simulink model "filter_t1"  (R2017a)
settings: Solver=VariableStepAuto  StartTime=0.0  StopTime=19  RelTol=1e-3
settings Model: Creator=Chaohua Zhao  LastModifiedBy=Chaohua Zhao

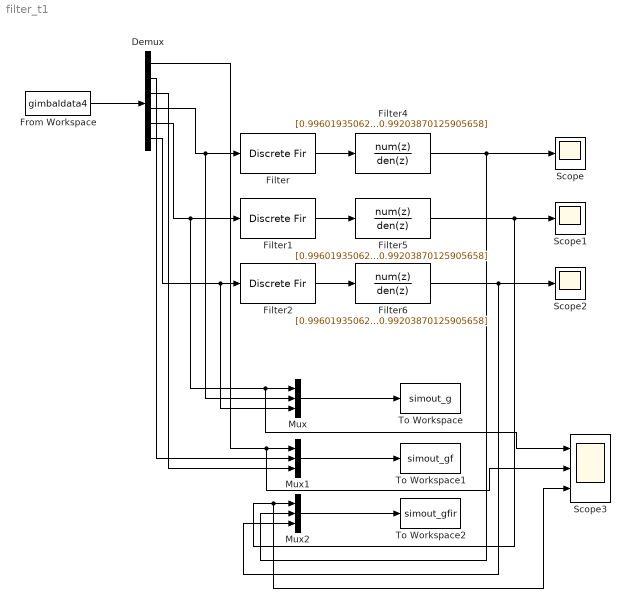
== system filter_t1 ==
  Demux : Demux  Outputs=6
  Filter : DiscreteFir  Tag=BlockMethodSubSystem  Coefficients=[6.3171406458817249e-18 0.038757485800321609 0.085067928451757008 0.12917070559097471 0.16083305039150533 0.17234165953088285 0.16083305039150533 0.12917070559097471 0.085067928451757008 0.038757485800321609 6.3171406458817249e-18]  InputProcessing=Columns as channels (frame based)
  Filter1 : DiscreteFir  Tag=BlockMethodSubSystem  Coefficients=[6.3171406458817249e-18 0.038757485800321609 0.085067928451757008 0.12917070559097471 0.16083305039150533 0.17234165953088285 0.16083305039150533 0.12917070559097471 0.085067928451757008 0.038757485800321609 6.3171406458817249e-18]  InputProcessing=Columns as channels (frame based)
  Filter2 : DiscreteFir  Tag=BlockMethodSubSystem  Coefficients=[6.3171406458817249e-18 0.038757485800321609 0.085067928451757008 0.12917070559097471 0.16083305039150533 0.17234165953088285 0.16083305039150533 0.12917070559097471 0.085067928451757008 0.038757485800321609 6.3171406458817249e-18]  InputProcessing=Columns as channels (frame based)
  Filter4 : DiscreteFilter  Tag=BlockMethodSubSystem  Numerator=[0.99601935062952829 -1.8886556848759783 0.99601935062952829]  Denominator=[1 -1.8886556848759783 0.99203870125905658]  InputProcessing=Columns as channels (frame based)  a0EqualsOne=on
  Filter5 : DiscreteFilter  Tag=BlockMethodSubSystem  Numerator=[0.99601935062952829 -1.8886556848759783 0.99601935062952829]  Denominator=[1 -1.8886556848759783 0.99203870125905658]  InputProcessing=Columns as channels (frame based)  a0EqualsOne=on
  Filter6 : DiscreteFilter  Tag=BlockMethodSubSystem  Numerator=[0.99601935062952829 -1.8886556848759783 0.99601935062952829]  Denominator=[1 -1.8886556848759783 0.99203870125905658]  InputProcessing=Columns as channels (frame based)  a0EqualsOne=on
  From Workspace : FromWorkspace  VariableName=gimbaldata4  SampleTime=0.001  OutputAfterFinalValue=Setting to zero
  Mux : Mux  Inputs=3
  Mux1 : Mux  Inputs=3
  Mux2 : Mux  Inputs=3
  Scope : Scope
  Scope1 : Scope
  Scope2 : Scope
  Scope3 : Scope  NumInputPorts=3
  To Workspace : ToWorkspace  VariableName=simout_g  SampleTime=-1
  To Workspace1 : ToWorkspace  VariableName=simout_gf  SampleTime=-1
  To Workspace2 : ToWorkspace  VariableName=simout_gfir  SampleTime=-1
  wires:
  From Workspace/1 -> Demux/1
  Demux/4 -> Mux/2, Filter/1
  Demux/5 -> Scope3/1, Mux/1, Filter1/1
  Demux/6 -> Mux/3, Filter2/1
  Filter/1 -> Filter4/1
  Filter1/1 -> Filter5/1
  Filter2/1 -> Filter6/1
  Mux/1 -> To Workspace/1
  Demux/1 -> Scope3/2, Mux1/1
  Demux/2 -> Mux1/2
  Demux/3 -> Mux1/3
  Mux1/1 -> To Workspace1/1
  Mux2/1 -> To Workspace2/1
  Filter4/1 -> Mux2/2, Scope/1
  Filter5/1 -> Scope3/3, Mux2/1, Scope1/1
  Filter6/1 -> Mux2/3, Scope2/1
